simulink model "RTS_8km"  (R2018a)
settings: Solver=FixedStepAuto  StartTime=0.0  StopTime=10  FixedStep=Ts  MaxStep=Ts  RelTol=1e-3  AbsTol=1e-6
values from neighbouring files (symbols this model uses):
  Cline = v*inv(M)*C1    [DynamicModelParameters.m]
  Kline = inv(M)*(g*K0+v^2*K2)    [DynamicModelParameters.m]
  Mline = inv(M)    [DynamicModelParameters.m]
  sysDC = c2d(sysC,Ts)    [DynamicModelParameters.m]
  sysDi = c2d(sysi, Ts)    [DynamicModelParameters.m]
  sysDo = c2d(syso, Ts)    [DynamicModelParameters.m]
  sysDW = c2d(sysW, Ts)    [DynamicModelParameters.m]
libraries: simulink x3, simulink_extras x2
settings Model: Creator=FoR  LastModifiedBy=gct14001
settings SolverCC: SolverResetMethod=Robust
settings CodeAppCC: StateflowObjectComments=on

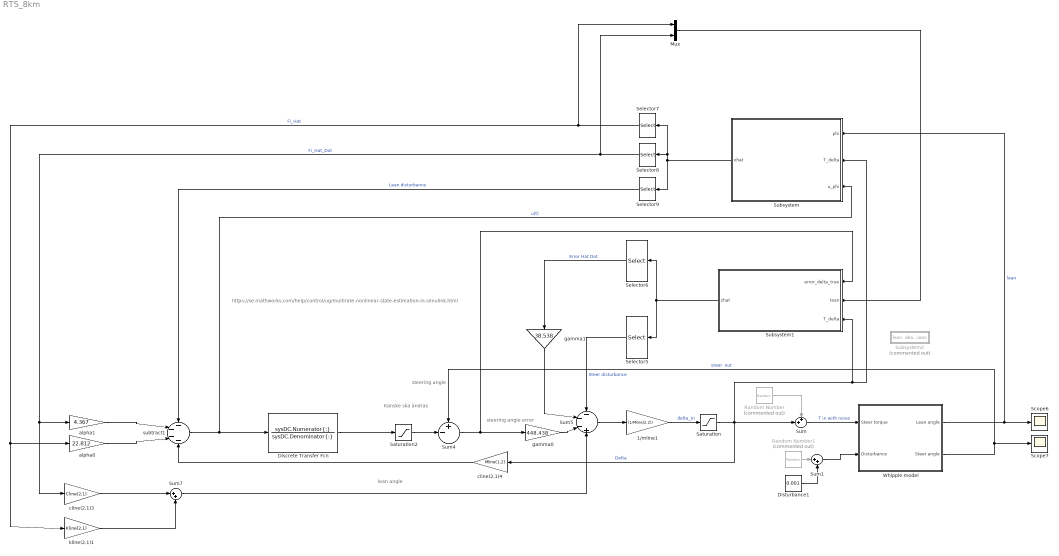
== system RTS_8km ==
  note: steering angle
  note: https://se.mathworks.com/help/control/ug/multirate-nonlinear-state-estimation-in-simulink.html
  note: steering angle error
  note: Kanske ska
      | ändras
  note: lean angle
  1/mline1 : Gain  Gain=(1/Mline(2,2))
  Discrete Transfer Fcn : DiscreteTransferFcn  Numerator=sysDC.Numerator{:}  Denominator=sysDC.Denominator{:}
  Disturbance1 : Constant  Value=0.001
  Mux : Mux  Inputs=2
  Random Number : RandomNumber  Commented=on  Variance=0.1  SampleTime=0.1
  Random Number1 : RandomNumber  Commented=on  Variance=0.1  SampleTime=0.1
  Saturation : Saturate  UpperLimit=12  LowerLimit=-12
  Saturation2 : Saturate  UpperLimit=pi/2  LowerLimit=-pi/2
  Scope6 : Scope
  Scope7 : Scope
  Selector5 : Selector  InputPortWidth=6  IndexOptions=Index vector (dialog)  Indices=3  OutputSizes=1
  Selector6 : Selector  InputPortWidth=6  IndexOptions=Index vector (dialog)  Indices=2  OutputSizes=1
  Selector7 : Selector  InputPortWidth=3  IndexOptions=Index vector (dialog)  Indices=1  OutputSizes=1
  Selector8 : Selector  InputPortWidth=3  IndexOptions=Index vector (dialog)  Indices=2  OutputSizes=1
  Selector9 : Selector  InputPortWidth=3  IndexOptions=Index vector (dialog)  Indices=3  OutputSizes=1
  Subsystem : Subsystem
  Subsystem1 : Subsystem
  Subsystem2 : Subsystem  Commented=on
  Sum : Sum  Inputs=++|
  Sum1 : Sum  Inputs=|++
  Sum4 : Sum  Inputs=+-|
  Sum5 : Sum  Inputs=---+
  Sum7 : Sum  Inputs=|++
  Whipple model : Subsystem
  alpha0 : Gain  Gain=22.812
  alpha1 : Gain  Gain=4.367
  cline(2,1)3 : Gain  Gain=Cline(2,1)
  cline(2,1)4 : Gain  Gain=Mline(1,2)
  gamma0 : Gain  Gain=448.438
  "gamma1 " : Gain  Gain=38.538
  kline(2,1)1 : Gain  Gain=Kline(2,1)
  subtract1 : Sum  Inputs=----
  wires:
  Saturation/1 -> Sum/2, cline(2,1)4/1, Subsystem1/3(T_delta), Subsystem/2(T_delta)  "Delta"
  Subsystem1/1(zhat) -> Selector5/1, Selector6/1
  Selector7/1 -> Mux/1, kline(2,1)1/1, alpha0/1  "Fi_Hat"
  cline(2,1)3/1 -> Sum7/1
  Selector9/1 -> subtract1/1  "Lean disturbance"
  cline(2,1)4/1 -> subtract1/4
  Selector5/1 -> Sum5/1  "Steer disturbance"
  Sum7/1 -> Sum5/4
  Sum5/1 -> 1/mline1/1
  alpha0/1 -> subtract1/3
  alpha1/1 -> subtract1/2
  gamma0/1 -> Sum5/3
  kline(2,1)1/1 -> Sum7/2
  subtract1/1 -> Discrete Transfer Fcn/1, Subsystem/3(u_phi)  "u(t)"
  1/mline1/1 -> Saturation/1  "delta_In"
  Selector8/1 -> Mux/2, cline(2,1)3/1, alpha1/1  "Fi_Hat_Dot"
  "gamma1 "/1 -> Sum5/2
  Sum4/1 -> Subsystem1/1(error_delta_true), gamma0/1
  Selector6/1 -> "gamma1 "/1  "Error Hat Dot"
  Saturation2/1 -> Sum4/2
  Subsystem/1(xhat) -> Selector8/1, Selector7/1, Selector9/1
  Whipple model/2(Steer angle) -> Sum4/1, Scope7/1  "steer  out"
  Discrete Transfer Fcn/1 -> Saturation2/1
  Sum/1 -> Whipple model/1(Steer torque)  "T in with noise"
  Random Number/1 -> Sum/1
  Whipple model/1("Lean angle ") -> Scope6/1, Subsystem/1(phi)  "lean"
  Sum1/1 -> Whipple model/2(Disturbance)
  Random Number1/1 -> Sum1/1
  Disturbance1/1 -> Sum1/2
  Mux/1 -> Subsystem1/2(lean)

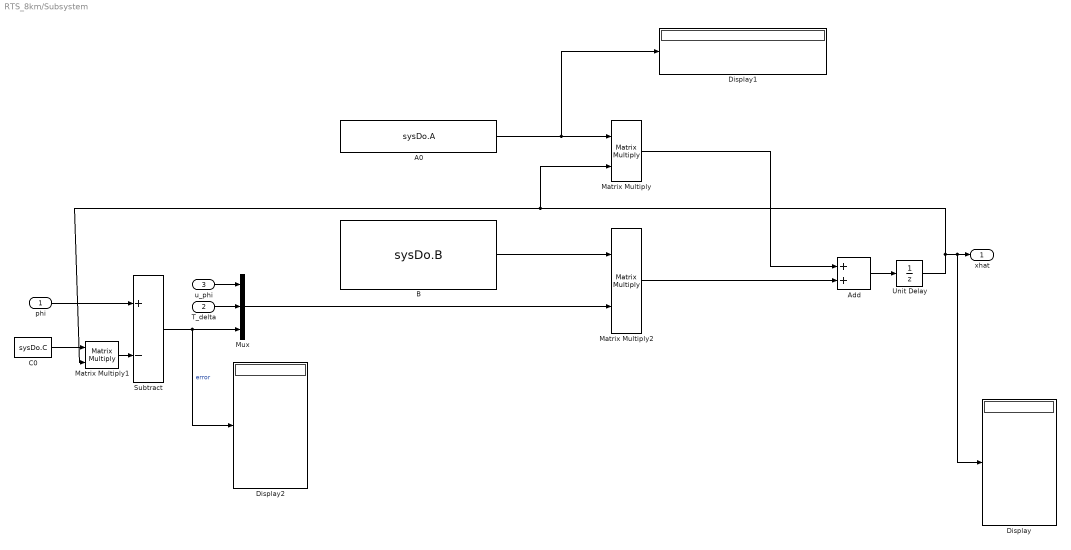
== system RTS_8km/Subsystem ==
  phi : Inport
  T_delta : Inport  Port=2
  u_phi : Inport  Port=3
  A0 : Constant  Value=sysDo.A
  Add : Sum
  B : Constant  Value=sysDo.B  VectorParams1D=off
  C0 : Constant  Value=sysDo.C  VectorParams1D=off
  Display : Display
  Display1 : Display
  Display2 : Display
  Matrix Multiply : Product  Multiplication=Matrix(*)
  Matrix Multiply1 : Product  Multiplication=Matrix(*)
  Matrix Multiply2 : Product  Multiplication=Matrix(*)
  Mux : Mux  Inputs=3
  Subtract : Sum  Inputs=+-
  Unit Delay : UnitDelay  SampleTime=-1
  xhat : Outport
  wires:
  A0/1 -> Display1/1, Matrix Multiply/1
  C0/1 -> Matrix Multiply1/1
  Matrix Multiply1/1 -> Subtract/2
  phi/1 -> Subtract/1
  Matrix Multiply/1 -> Add/1
  Matrix Multiply2/1 -> Add/2
  Add/1 -> Unit Delay/1
  Unit Delay/1 -> Display/1, xhat/1, Matrix Multiply1/2, Matrix Multiply/2
  B/1 -> Matrix Multiply2/1
  T_delta/1 -> Mux/2
  u_phi/1 -> Mux/1
  Subtract/1 -> Display2/1, Mux/3  "error"
  Mux/1 -> Matrix Multiply2/2

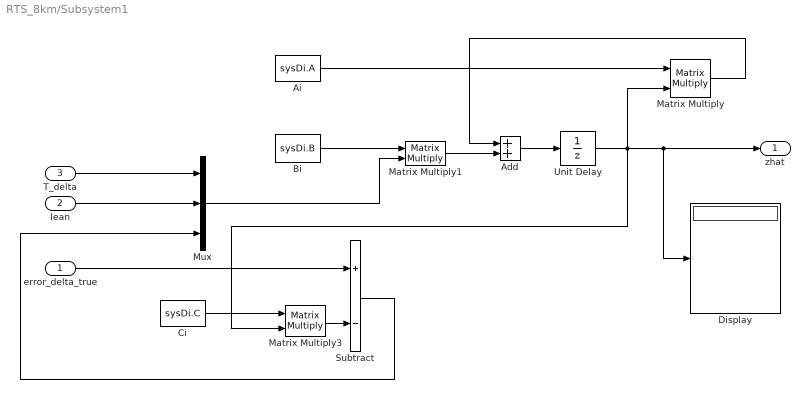
== system RTS_8km/Subsystem1 ==
  error_delta_true : Inport
  lean : Inport  Port=2
  T_delta : Inport  Port=3
  Add : Sum
  Ai : Constant  Value=sysDi.A
  "Bi " : Constant  Value=sysDi.B  VectorParams1D=off
  Ci : Constant  Value=sysDi.C  VectorParams1D=off
  Display : Display
  Matrix Multiply : Product  Multiplication=Matrix(*)
  Matrix Multiply1 : Product  Multiplication=Matrix(*)
  Matrix Multiply3 : Product  Multiplication=Matrix(*)
  Mux : Mux  Inputs=3
  Subtract : Sum  Inputs=+-
  Unit Delay : UnitDelay  SampleTime=-1
  zhat : Outport
  wires:
  Ai/1 -> Matrix Multiply/1
  Matrix Multiply/1 -> Add/1
  Matrix Multiply1/1 -> Add/2
  Ci/1 -> Matrix Multiply3/1
  error_delta_true/1 -> Subtract/1
  Matrix Multiply3/1 -> Subtract/2
  Add/1 -> Unit Delay/1
  Unit Delay/1 -> Matrix Multiply/2, Matrix Multiply3/2, Display/1, zhat/1
  lean/1 -> Mux/2
  T_delta/1 -> Mux/1
  "Bi "/1 -> Matrix Multiply1/1
  Subtract/1 -> Mux/3
  Mux/1 -> Matrix Multiply1/2

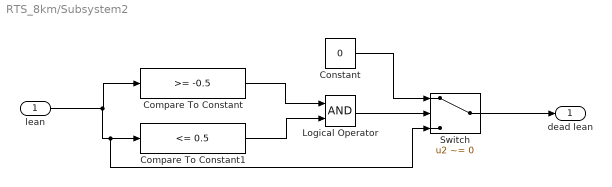
== system RTS_8km/Subsystem2 ==
  lean : Inport
  Compare To Constant : simulink/Logic and Bit Operations/Compare To Constant  relop=>=  const=-0.5  OutDataTypeStr=boolean
  Compare To Constant1 : simulink/Logic and Bit Operations/Compare To Constant  relop=<=  const=0.5  OutDataTypeStr=boolean
  Constant : Constant  Value=0
  Logical Operator : Logic  AllPortsSameDT=off  OutDataTypeStr=boolean
  Switch : Switch  Criteria=u2 ~= 0
  dead lean : Outport
  wires:
  Switch/1 -> dead lean/1
  Compare To Constant1/1 -> Logical Operator/2
  lean/1 -> Switch/3, Compare To Constant1/1, Compare To Constant/1
  Logical Operator/1 -> Switch/2
  Compare To Constant/1 -> Logical Operator/1
  Constant/1 -> Switch/1

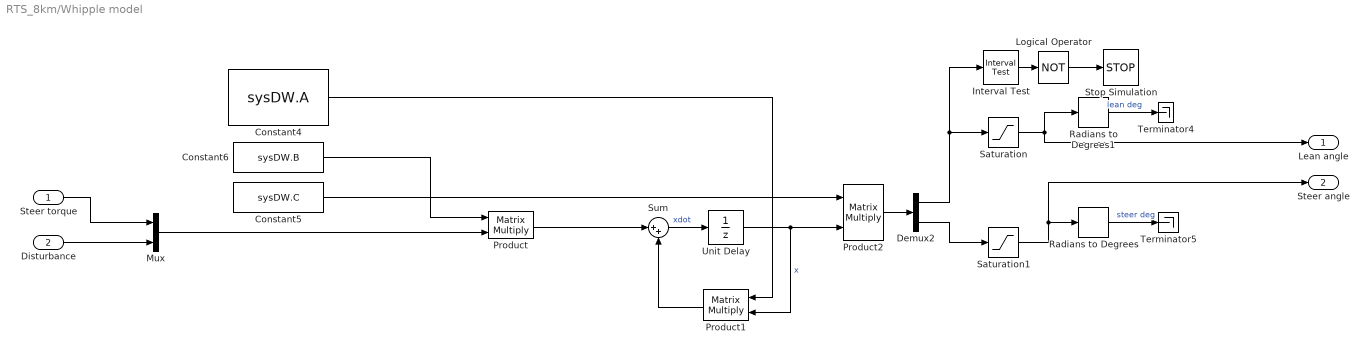
== system RTS_8km/Whipple model ==
  Steer torque : Inport
  Disturbance : Inport  Port=2
  Constant4 : Constant  Value=sysDW.A
  Constant5 : Constant  Value=sysDW.C
  Constant6 : Constant  Value=sysDW.B
  Demux2 : Demux  Outputs=2
  Interval Test : simulink/Logic and Bit Operations/Interval Test  IntervalClosedRight=on  uplimit=pi/4  IntervalClosedLeft=on  lowlimit=-pi/4  OutDataTypeStr=boolean
  Logical Operator : Logic  Operator=NOT  AllPortsSameDT=off  OutDataTypeStr=boolean
  Mux : Mux  Inputs=2
  Product : Product  Multiplication=Matrix(*)
  Product1 : Product  Multiplication=Matrix(*)
  Product2 : Product  Multiplication=Matrix(*)
  Radians to Degrees : simulink_extras/Transformations/Radians to Degrees
  Radians to Degrees1 : simulink_extras/Transformations/Radians to Degrees
  Saturation : Saturate  UpperLimit=pi/2  LowerLimit=-pi/2
  Saturation1 : Saturate  UpperLimit=pi/2  LowerLimit=-pi/2
  Stop Simulation : Stop
  Sum : Sum  Inputs=|++
  Terminator4 : Terminator
  Terminator5 : Terminator
  Unit Delay : UnitDelay  SampleTime=-1
  "Lean angle " : Outport
  Steer angle : Outport  Port=2
  wires:
  Saturation/1 -> "Lean angle "/1, Radians to Degrees1/1
  Saturation1/1 -> Steer angle/1, Radians to Degrees/1
  Demux2/1 -> Interval Test/1, Saturation/1
  Product1/1 -> Sum/2
  Constant6/1 -> Product/1
  Demux2/2 -> Saturation1/1
  Radians to Degrees1/1 -> Terminator4/1  "lean deg"
  Sum/1 -> Unit Delay/1  "xdot"
  Product/1 -> Sum/1
  Interval Test/1 -> Logical Operator/1
  Product2/1 -> Demux2/1
  Unit Delay/1 -> Product1/2, Product2/2  "x"
  Logical Operator/1 -> Stop Simulation/1
  Constant4/1 -> Product1/1
  Constant5/1 -> Product2/1
  Radians to Degrees/1 -> Terminator5/1  "steer deg"
  Disturbance/1 -> Mux/2
  Steer torque/1 -> Mux/1
  Mux/1 -> Product/2
